simulink model "modelo_3"  (R2020a)
settings: Solver=VariableStepAuto  StartTime=0.0  StopTime=259200  RelTol=1e-3
values from neighbouring files (symbols this model uses):
  p = exp(DE/T)    [s_annealing.m]
  Pnom = 2e6    (= 2000000)    [Parametros.m]
  Pnom1 = 2e6    (= 2000000)    [Parametros.m]
  w_max = 26    [Parametros.m]
  w_min = 6    [Parametros.m]
undefined symbols (not defined in the file or in its folder): F, find_system, Fnom, gcbh, H, Llr, Lls, Rr, Rs, sps_rtmsupport, Vnom, Wind_On
libraries: powerlib x12, powerlib_meascontrol x2, re_lib x1
settings Model: Creator=octad  LastModifiedBy=octad

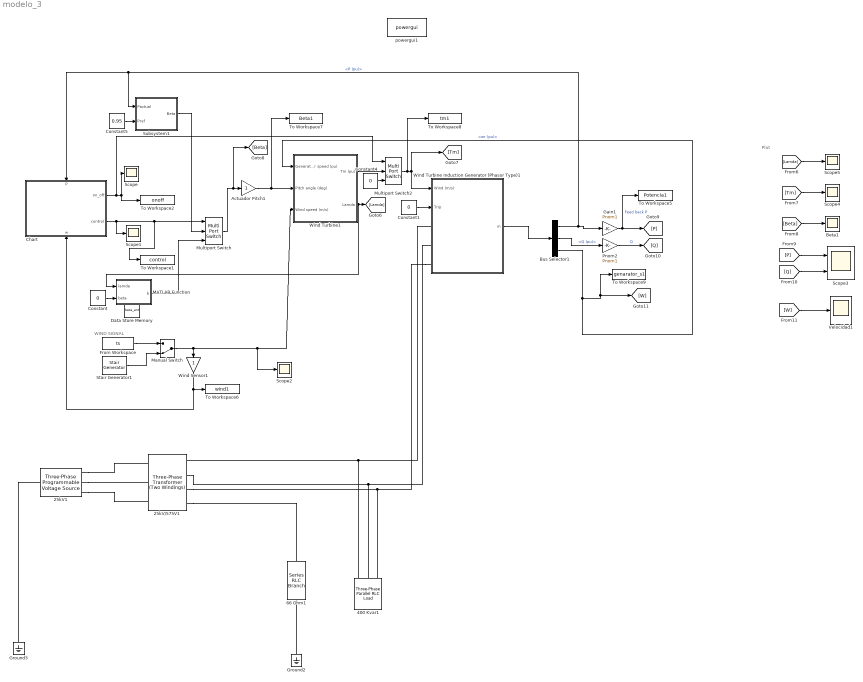
== system modelo_3 ==
  note: WIND SIGNAL
  note: Plot
  25kV/575V1 : powerlib/Elements/Three-Phase Transformer (Two Windings)  Winding1Connection=Yg  Winding2Connection=Yn  CoreType=Three single-phase transformers  SetSaturation=off  Hysteresis=off  DataFile='hysteresis'  SetInitialFlux=off  Measurements=None  UNITS=pu  NominalPower=[ 4e6 , 60 ]  Winding1=[ 25e3 , 0.025/30 , 0.025]  Winding2=[575 , 0.025/30 , 0.025 ]  Rm=500  Lm=inf  L0=0.5  Saturation=[ 0,0 ; 0.0024,1.2 ; 1.0,1.52 ]  InitialFluxes=[ 0.8 , -0.8 , 0.7 ]  BreakLoop=off  DiscreteSolver=Trapezoidal iterative  DataType=off  TransfoNumber=1
  25kV1 : powerlib/Electrical Sources/Three-Phase Programmable Voltage Source  PositiveSequence="[25000  0 60]"  VariationEntity=None  VariationType=Table of time-amplitude pairs  VariationTypeAlt=Step  VariationStep=0.5  VariationRate=10  VariationMagnitude=0.3  VariationFrequency=2  VariationTiming=[1 2]  VariationPhaseA=off  Amplitudes=[1 0.8 1.2 1.0]  TimeValues=[0 0.1 0.15 0.2]  HarmonicGeneration=off  HarmonicA=[3 0.2 -25 0]  HarmonicB=[2 0.15 35 2]  Timing="[0.05  3]"  BusType=swing  Pref=0  Qref=0  Qmin=-inf  Qmax=inf
  400 Kvar1 : powerlib/Elements/Three-Phase Parallel RLC Load  LConnTagsString=A|B|C  Configuration=Delta  NominalVoltage=575  Vabc=[1e3 1e3 1e3]  Vabcp=[1e3 1e3 1e3]  NominalFrequency=60  UnbalancedPower=off  ActivePower=0  InductivePower=0  CapacitivePower=400e3  Pabc=[10e3 9e3 11e3]  QLabc=[100 90 110]  QCabc=[100 90 110]  Pabcp=[10e3 9e3 11e3]  QLabcp=[100 90 110]  QCabcp=[100 90 110]  Measurements=None  LoadType=constant Z
  66 Ohm1 : powerlib/Elements/Series RLC Branch  LConnTagsString=__new0  RConnTagsString=__new0  BranchType=R  Resistance=66  Inductance=1e-3  SetiL0=off  InitialCurrent=0  Capacitance=1e-6  Setx0=off  InitialVoltage=0  Measurements=None
  Actuador Pitch1 : Gain
  Beta1 : Scope
  Bus Selector1 : BusSelector  OutputSignals=P (pu),Q (pu),wr (pu)
  Chart : Stateflow chart  TreatAsAtomicUnit=on
      settings: PortSchema="{\"entries\":[{\"content\":{\"sides\":[{\"content\":{\"connectorIds\":[]},\"type\":\"ConnectorPlacement.EquallySpacedRectSide\",\"uuid\":\"76455593-48be-4327-99eb-22cda1041c6c\"},{\"content\":{\"connectorIds\":[\"Out1\",\"Out2\"],\"side\":\"RIGHT\"},\"type\":\"ConnectorPlacement.EquallySpacedRectSide\",\"uuid\":\"0938c4e6-de83-48e5-b141-0954c3497832\"},{\"content\":{\"connectorIds\":[\"In2\"],\"side\":\"TOP\"},\"type\":\"ConnectorPlacement.EquallySpacedRectSide\",\"uuid\":\"886ddab1-e8c7-4b68-9a93-78c994632caa\"},{\"content\":{\"connectorIds\":[\"In1\"],\"side\":\"BOTTOM\"},\"type\":\"ConnectorPlacement.EquallySpacedRectSide\",\"uuid\":\"6af41394-77cd-4861-af48-a316959a0c75\"}]},\"type\":\"ConnectorPlacement.EquallySpacedConnector\",\"uuid\":\"704104a5-98c5-46da-8d41-4491e31041ef\"}],\"packageUris\":[\"http://schema.mathworks.com/mf0/Connector/19700101\"],\"version\":\"1.0\"}"
  Constant : Constant  Value=0
  Constant1 : Constant  Value=0
  Constant4 : Constant  Value=0
  Constant5 : Constant  Value=0.95
  Data Store Memory : DataStoreMemory  DataStoreName=beta_ant  ReadBeforeWriteMsg=warning  WriteAfterWriteMsg=warning  WriteAfterReadMsg=warning  ShowAdditionalParam=off  OutDataTypeStr=double
  From Workspace : FromWorkspace  VariableName=ts
  Gain1 : Gain  Gain=Pnom1
  Ground2 : powerlib/Elements/Ground  LConnTagsString=a
  Ground3 : powerlib/Elements/Ground  LConnTagsString=a
  MATLAB Function : MATLAB Function  TreatAsAtomicUnit=on
  Manual Switch : ManualSwitch  CurrentSetting=0
  Multiport Switch : MultiPortSwitch  DataPortOrder=Specify indices  Inputs=2  DataPortIndices={1,2}  DiagnosticForDefault=None
  Multiport Switch2 : MultiPortSwitch  DataPortOrder=Specify indices  Inputs=2  DataPortIndices={1,2}  DiagnosticForDefault=None
  Pnom2 : Gain  Gain=Pnom1
  Scope{,1..2,4..5} (5 alike) : Scope
  Scope3 : Scope  NumInputPorts=2
  Stair Generator1 : powerlib_meascontrol/Pulse & Signal Generators/Stair Generator  t=time  e=wind_d  Ts=100
  Subsystem1 : Subsystem
  To Workspace1 : ToWorkspace  VariableName=control  SaveFormat=Timeseries  SampleTime=-1
  To Workspace2 : ToWorkspace  VariableName=onoff  SaveFormat=Timeseries  SampleTime=-1
  To Workspace5 : ToWorkspace  VariableName=Potencia1  SaveFormat=Timeseries  SampleTime=-1
  To Workspace6 : ToWorkspace  VariableName=wind1  SaveFormat=Timeseries  SampleTime=-1
  To Workspace7 : ToWorkspace  VariableName=Beta1  SaveFormat=Timeseries  SampleTime=-1
  To Workspace8 : ToWorkspace  VariableName=tm1  SaveFormat=Timeseries  SampleTime=-1
  To Workspace9 : ToWorkspace  VariableName=genarator_s1  SaveFormat=Timeseries  SampleTime=-1
  Velocidad1 : Scope
  Wind Sensor1 : Gain
  Wind Turbine Induction Generator (Phasor Type)1 : Subsystem  AncestorBlock=|  DialogController=POWERSYS.PowerSysDialog  LoadFcn=sps_rtmsupport('LoadFcn',gcbh); %find_system(gcs,'FollowLinks', 'on', 'LookUnderMasks', 'all');  StartFcn=sps_rtmsupport('StartFcn',gcbh);  StopFcn=sps_rtmsupport('StopFcn',gcbh);  mask(Wind Turbine Induction Generator (Phasor Type)){ExternalTm=on, nom=[Pnom1/0.9, 575, 60], sta=[ 0.004843, 0.1248], rot=[ 0.004377, 0.1791], Lm=6.77, mec=[5.04, 0.01, 3], init=[ -0.01,0,   0,0,0,   0,0,0 ], pitch_angle=0, Pmec=1.5e6, wind_base=12, speed_nom=1, P_wind_base=1, K_pitch_gain=[5 25], pitch_max=45, pitch_rate=2}
      | re_lib/Wind Generation/Wind Turbine
      | Induction Generator
      | (Phasor Type)
      mask prompts: ExternalTm "External turbine (Tm mechanical torque input)"; nom "Nominal power, line-to-line voltage, frequency [Pn(VA), Vn(Vrms), fn(Hz)]:"; sta "Stator [Rs, Lls] (pu):"; rot "Rotor [Rr', Llr'] (pu):"; Lm "Magnetizing inductance Lm (pu):"; mec "Inertia constant, friction factor, and pairs of poles: [H(s), F(pu), p]"; init "Initial conditions [s, th(deg), ias, ibs, ics (pu), ph_as, ph_bs, ph_cs (pu)]:"; pitch_angle "Pitch angle beta used to display characteristics (beta >=0)  (deg):"; Pmec "Nominal wind turbine mechanical output power (W):"; wind_base "Base wind speed (m/s):"; speed_nom "Base rotational speed (pu of base generator speed):"; P_wind_base "Maximum power at base wind speed (pu of nominal mechanical power):"; K_pitch_gain "Pitch angle controller gain: [Kp Ki]"; pitch_max "Maximum pitch angle (deg):"; pitch_rate "Maximum rate of change of pitch angle (deg/s):"
      mask help: Implements a phasor model of a squirrel-cage induction generator driven by a wind turbine.
      mask init:
      | [Pnom,Vnom,Fnom,Rs,Lls,Rr,Llr,H,p,F,Wind_On,FACTSroot] = WindTurbineIndGenInit (nom,sta,rot,mec,ExternalTm,wind_base,gcbh);
      settings: CopyFcn=sps_rtmsupport('CopyFcn',gcbh);  DeleteFcn=sps_rtmsupport('DeleteFcn',gcbh);  UndoDeleteFcn=sps_rtmsupport('UndoDeleteFcn',gcbh);  ModelCloseFcn=sps_rtmsupport('ModelCloseFcn',gcbh);  PreSaveFcn=sps_rtmsupport('PreSaveFcn',gcbh);  PostSaveFcn=sps_rtmsupport('PostSaveFcn',gcbh);  NameChangeFcn=sps_rtmsupport('NameChangeFcn',gcbh);  PreCopyFcn=sps_rtmsupport('PreCopyFcn',gcbh);  OpenFcn=sps_rtmsupport('OpenFcn',gcbh, [1]);  CloseFcn=sps_rtmsupport('CloseFcn',gcbh);  PreDeleteFcn=sps_rtmsupport('PreDeleteFcn',gcbh);
      mask Help: helpview(psbhelp);
      mask Callback ExternalTm: WindTurbineIndGenCback(gcbh);
      mask DialogControl generatordata Prompt: Generator
      mask DialogControl Turbine Prompt: Turbine
      mask DialogControl display Prompt: Display wind turbine power characteristics
      mask DialogControl display Callback: WindTurbineIndGenDisplay(gcbh);
      mask Display:
      | image(imread(fullfile(FACTSroot,'eolienne.bmp'),'bmp'))
      | color('white')
      | port_label('LConn',1,'A')
      | port_label('LConn',2,'B')
      | port_label('LConn',3,'C')
      | color('blue')
      | port_label('output',1,'m')
      | switch get_param(gcbh,'ExternalTm')
      |     case 'on'
      |         port_label('input',1,'Tm')
      |     case 'off'
      |         port_label('input',1,'wind')
      | end
      | port_label('input',2,'trip')
  Wind Turbine1 : Subsystem  AncestorBlock=re_lib/Wind Generation/Wind Turbine  DialogController=POWERSYS.PowerSysDialog  mask(Wind Turbine){Pnom=Pnom, Pelec_base=Pnom1/0.9, wind_base=7.55, P_wind_base=0.5, speed_nom=1, pitch_angle=0, c1_c6=[0.51763          116          0.4            5           21     0.006795], cp_nom=0.48, lambda_nom=8.1}
      mask prompts: Pnom "Nominal mechanical output power (W):"; Pelec_base "Base power of the electrical generator (VA):"; wind_base "Base wind speed (m/s):"; P_wind_base "Maximum power at base wind speed (pu of nominal mechanical power):"; speed_nom "Base rotational speed (p.u. of base generator speed):"; pitch_angle "Pitch angle beta to display wind-turbine power characteristics (beta >=0)  (deg):"
      mask help:
      | This block implements a variable pitch wind turbine model. The performance coefficient Cp of the turbine is the mechanical output power of the turbine divided by wind power and a function of wind speed, rotational speed, and pitch angle (beta). Cp reaches its maximum value at zero beta. Select the wind-turbine power characteristics display to plot the turbine characteristics at the specified pitch angle.
      |
      | The first input is the generator speed in per unit of the generator base speed. For a synchronous or asynchronous generator, the base speed is the synchronous speed. For a permanent-magnet generator, the base speed is defined as the speed producing nominal voltage at  no load. The second input is the blade pitch angle (beta) in degrees. The third input is the wind speed in m/s.
      |
      | The output is the torque applied to the generator shaft in per unit of the generator ratings.
      |
      | The turbine inertia must be added to the generator inertia.
      mask init:
      | c1=c1_c6(1);c2=c1_c6(2);c3=c1_c6(3);c4=c1_c6(4);c5=c1_c6(5);c6=c1_c6(6);
      | 
      | if Pnom<=0
      |     error(message('physmod:powersys:common:GreaterThan',getfullname(gcbh),'Nominal mechanical output power',0));
      | end
      | if Pelec_base<=0
      |     error(message('physmod:powersys:common:GreaterThan',getfullname(gcbh),'Base power of the electrical generator',0));
      | end
      | if wind_base<=0
      |     error(message('physmod:powersys:common:GreaterThan',getfullname(gcbh),'Base wind speed (m/s)',0));
      | end
      | if P_wind_base<=0
      |     error(message('physmod:powersys:common:GreaterThan',getfullname(gcbh),'Maximum power at base wind speed',0));
      | end
      | power_initmask();
      settings: OpenFcn=sps_rtmsupport('OpenFcn',gcbh)
      mask Help: helpview(psbhelp);
      mask DialogControl DisplayTurbChar Prompt: Display wind turbine power characteristics
      mask DialogControl DisplayTurbChar Callback: WindTurbinePlot(gcb)
      mask Display: disp('');
  powergui1 : powerlib/powergui  Priority=1  SimulationMode=Phasor  SampleTime=50e-6  frequency=60  Iterations=50  frequencyindice=60  Pbase=100e6  ErrMax=1e-4  UnitsV=kV  UnitsW=MW  buscounter=0  FunctionMessages=off  echomessages=off  EnableUseOfTLC=off  CurrentSourceSwitches=off  DisableSnubberDevices=off  DisableRonSwitches=off  DisableVfSwitches=off  DisplayEquations=off  AutomaticDiscreteSolvers=off  SolverType=Tustin/Backward Euler (TBE)  Interpol=off  ExternalGateDelay=off  methode=off  Ts=100  x0status=blocks  SPID=on  SwTol=0  HookPort=off  NonlinearTolerance=1e-4  nMaxIteration=100  ContinueOnMaxIteration=off  RestoreLinks=warning  ResistiveCurrentMeasurement=off  Frange=[0:2:500]  Ylog=off  Xlog=on  ShowGrid=off  save=off  variable=ZData  structure=0  ZoomFFT=off  StartTime=0.0  cycles=1  DisplayStyle=1  fundamental=60  FreqAxis=off  MaxFrequency=1000  frequencyindicesteady=1  RmsSteady=1  display=off
  wires:
  Bus Selector1/1 -> Chart/2(P), Subsystem1/1(Pactual), Gain1/1  "<P (pu)>"
  Constant/1 -> MATLAB Function/2(beta)
  [Q] -> Scope3/2
  [Beta] -> Beta1/1
  Bus Selector1/2 -> Pnom2/1  "<Q (pu)>"
  Gain1/1 -> [P], To Workspace5/1  "Feed back P"
  Subsystem1/1(Beta) -> Multiport Switch/2
  Wind Turbine1/1(Tm (pu)) -> Multiport Switch2/2
  Wind Turbine Induction Generator (Phasor Type)1/1(m) -> Bus Selector1/1
  Pnom2/1 -> [Q]  "Q"
  Wind Sensor1/1 -> Chart/1(w), To Workspace6/1
  Wind Turbine1/2(Lamda) -> MATLAB Function/1(lamda), [Lamda]
  [P] -> Scope3/1
  Actuador Pitch1/1 -> To Workspace7/1, Wind Turbine1/2(Pitch angle (deg))
  [Lamda] -> Scope5/1
  [W] -> Velocidad1/1
  Constant5/1 -> Subsystem1/2(Pref)
  [Tm] -> Scope4/1
  Bus Selector1/3 -> [W], To Workspace9/1, Wind Turbine1/1(Generator speed (pu))  "<wr (pu)>"
  Multiport Switch/1 -> [Beta], Actuador Pitch1/1
  MATLAB Function/1(b) -> Multiport Switch/3
  Chart/2(control) -> Scope1/1, To Workspace1/1, Multiport Switch/1
  Chart/1(on_off) -> Multiport Switch2/1, Scope/1, To Workspace2/1
  Constant1/1 -> Wind Turbine Induction Generator (Phasor Type)1/2(Trip)
  Multiport Switch2/1 -> To Workspace8/1, [Tm], Wind Turbine Induction Generator (Phasor Type)1/1("Wind (m/s) ")
  Constant4/1 -> Multiport Switch2/3
  From Workspace/1 -> Manual Switch/1
  Stair Generator1/1 -> Manual Switch/2
  Manual Switch/1 -> Wind Sensor1/1, Scope2/1, Wind Turbine1/3(Wind speed (m/s))
  connections:
  400 Kvar1/LConn2 -- Wind Turbine Induction Generator (Phasor Type)1/LConn2 -- 25kV/575V1/RConn2
  Wind Turbine Induction Generator (Phasor Type)1/LConn3 -- 25kV/575V1/RConn3 -- 400 Kvar1/LConn3
  Wind Turbine Induction Generator (Phasor Type)1/LConn1 -- 25kV/575V1/RConn1 -- 400 Kvar1/LConn1
  25kV1/RConn1 -- 25kV/575V1/LConn1
  Ground2/LConn1 -- 66 Ohm1/RConn1
  Ground3/LConn1 -- 25kV1/LConn1
  25kV1/RConn2 -- 25kV/575V1/LConn2
  25kV/575V1/RConn4 -- 66 Ohm1/LConn1
  25kV1/RConn3 -- 25kV/575V1/LConn3

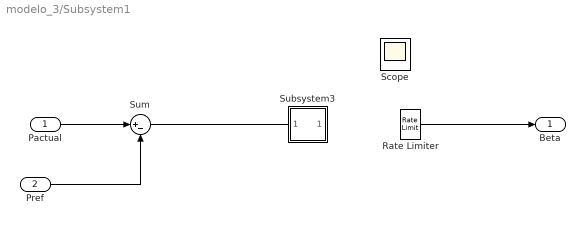
== system modelo_3/Subsystem1 ==
  Pactual : Inport
  Pref : Inport  Port=2
  "Rate Limiter   " : RateLimiter  RisingSlewLimit=2  FallingSlewLimit=-2
  Scope : Scope
  Subsystem3 : Subsystem  AncestorBlock=|  mask{Kp=1, Ki=3, Limits=[45 0], Init=0}
      | re_lib/Wind Generation/Wind Turbine
      | Induction Generator
      | (Phasor Type)/Subsystem3
      mask prompts: Kp "Proportional gain (Kp):"; Ki "Integral gain (Ki):"; Limits "Output limits [Upper Lower]:"; Init "Output initial value:"
      mask init:
      | Upper_Limit=Limits(1);
      | Lower_Limit=Limits(2);
      mask Display: disp('PI')
  Sum : Sum  Inputs=|+-
  Beta : Outport
  wires:
  Pref/1 -> Sum/2
  ? -> Scope/1, "Rate Limiter   "/1
  "Rate Limiter   "/1 -> Beta/1
  Pactual/1 -> Sum/1
  Sum/1 -> ?

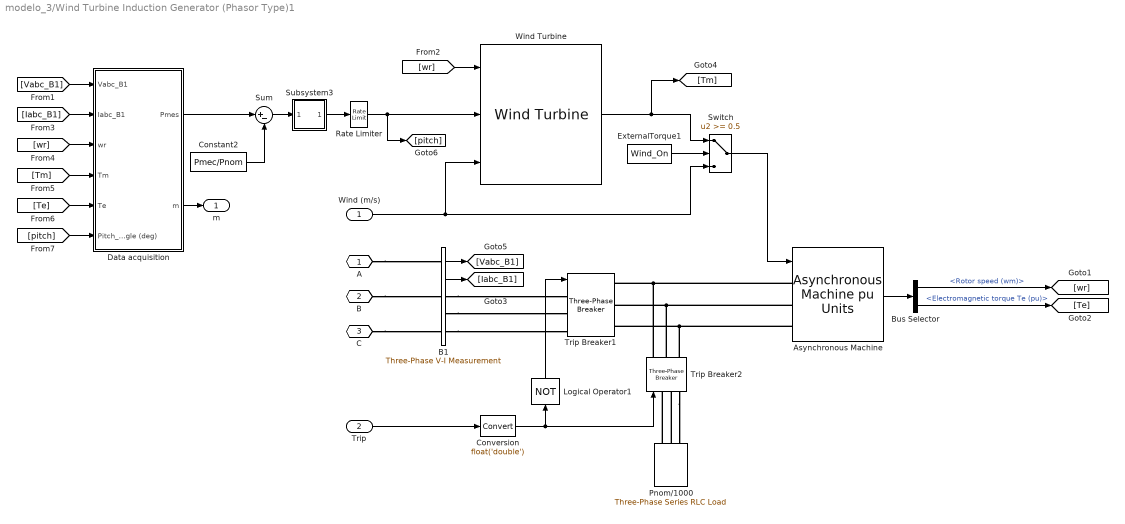
== system modelo_3/Wind Turbine Induction Generator (Phasor Type)1 ==
  "Wind (m/s) " : Inport
  Trip : Inport  Port=2
  Asynchronous Machine : powerlib/Machines/Asynchronous Machine pu Units  RotorType=Squirrel-cage  PresetModel=No  MechanicalLoad=Torque Tm  ShowDetailedParameters=on  ReferenceFrame=Rotor  Units=pu  MeasurementBus=off  NominalParameters=[ Pnom Vnom Fnom ]  Stator=[ Rs Lls]  Rotor=[ Rr Llr]  Cage1=[0.01909 0.0397]  Cage2=[0.01909 0.0397]  Lm=Lm  Mechanical=[H F p]  PolePairs=3  InitialConditions=init  SimulateSaturation=off  Saturation=[ 0 0 ; 0 0 ]  LoadFlowParameters=0  TsPowergui=0  TsBlock=-1  IterativeModel=Forward Euler  IterativeDiscreteModel=Trapezoidal non iterative  Pmec=0
      settings: SourceProductBaseCode=MT,PS
  B1 : powerlib/Measurements/Three-Phase V-I Measurement  VoltageMeasurement=phase-to-ground  SetLabelV=off  LabelV=Vabc_B1  Vpu=on  VpuLL=off  CurrentMeasurement=yes  SetLabelI=off  LabelI=Iabc_Beol  Ipu=on  Pbase=Pnom  Vbase=Vnom  OutputType=Complex  PhasorSimulation=on  PSBequivalent=0
      settings: SourceProductBaseCode=MT,PS
  Bus Selector : BusSelector  OutputSignals=Mechanical.Rotor speed (wm),Mechanical.Electromagnetic torque Te (pu)
  Constant2 : Constant  Value=Pmec/Pnom
  Conversion : DataTypeConversion  OutDataTypeStr=float('double')
  Data acquisition : Subsystem
  ExternalTorque1 : Constant  Value=Wind_On
  Logical Operator1 : Logic  Operator=NOT  AllPortsSameDT=off  OutDataTypeStr=float('double')  SampleTime=0
  Pnom/1000 : powerlib/Elements/Three-Phase Series RLC Load  LConnTagsString=A|B|C  Configuration=Y (grounded)  NominalVoltage=Vnom  Vabc=[1e3 1e3 1e3]  Vabcp=[1e3 1e3 1e3]  NominalFrequency=Fnom  UnbalancedPower=off  ActivePower=Pnom/1000  InductivePower=0  CapacitivePower=0  Pabc=[10e3 9e3 11e3]  QLabc=[100 90 110]  QCabc=[100 90 110]  Pabcp=[10e3 9e3 11e3]  QLabcp=[100 90 110]  QCabcp=[100 90 110]  Measurements=None  LoadType=constant Z
      settings: SourceProductBaseCode=MT,PS
  "Rate Limiter   " : RateLimiter  RisingSlewLimit=pitch_rate  FallingSlewLimit=-pitch_rate
  Subsystem3 : Subsystem  mask{Kp=K_pitch_gain(1), Ki=K_pitch_gain(2), Limits=[pitch_max 0], Init=0}
      mask prompts: Kp "Proportional gain (Kp):"; Ki "Integral gain (Ki):"; Limits "Output limits [Upper Lower]:"; Init "Output initial value:"
      mask init:
      | Upper_Limit=Limits(1);
      | Lower_Limit=Limits(2);
      mask Display: disp('PI')
  Sum : Sum  Inputs=|+-  SaturateOnIntegerOverflow=on
  Switch : Switch  Threshold=0.5  SaturateOnIntegerOverflow=on
  Trip Breaker1 : powerlib/Elements/Three-Phase Breaker  InitialState=closed  SwitchA=on  SwitchB=on  SwitchC=on  SwitchTimes="[4/60  10/60]"  External=on  BreakerResistance=0.001  SnubberResistance=1e6  SnubberCapacitance=inf  Measurements=None
      settings: SourceProductBaseCode=MT,PS
  Trip Breaker2 : powerlib/Elements/Three-Phase Breaker  InitialState=open  SwitchA=on  SwitchB=on  SwitchC=on  SwitchTimes="[4/60  10/60]"  External=on  BreakerResistance=0.001  SnubberResistance=1e6  SnubberCapacitance=inf  Measurements=None
      settings: SourceProductBaseCode=MT,PS
  Wind Turbine : re_lib/Wind Generation/Wind Turbine  Pnom=Pmec  Pelec_base=Pnom  wind_base=wind_base  P_wind_base=P_wind_base  speed_nom=speed_nom  pitch_angle=0  c1_c6="[0.51763          116          0.4            5           21     0.006795]"  cp_nom=0.48  lambda_nom=8.1
      settings: SourceProductBaseCode=PS
  A : PMIOPort  Side=Left
  B : PMIOPort  Port=2  Side=Left
  C : PMIOPort  Port=3  Side=Left
  m : Outport  VectorParamsAs1DForOutWhenUnconnected=off
  wires:
  Asynchronous Machine/1 -> Bus Selector/1
  Wind Turbine/1 -> Switch/1, [Tm]
  B1/2 -> [Iabc_B1]
  B1/1 -> [Vabc_B1]
  "Wind (m/s) "/1 -> Wind Turbine/3, Switch/3
  Data acquisition/2(m) -> m/1
  "Rate Limiter   "/1 -> Wind Turbine/2, [pitch]
  Bus Selector/1 -> [wr]  "<Rotor speed (wm)>"
  Bus Selector/2 -> [Te]  "<Electromagnetic torque Te (pu)>"
  [Iabc_B1] -> Data acquisition/2(Iabc_B1)
  [Vabc_B1] -> Data acquisition/1(Vabc_B1)
  [wr] -> Data acquisition/3(wr)
  [Tm] -> Data acquisition/4(Tm)
  [Te] -> Data acquisition/5(Te)
  [pitch] -> Data acquisition/6(Pitch_angle (deg))
  Trip/1 -> Conversion/1
  ExternalTorque1/1 -> Switch/2
  Switch/1 -> Asynchronous Machine/1
  Sum/1 -> Subsystem3/1(In1)
  Subsystem3/1(Out1) -> "Rate Limiter   "/1
  Constant2/1 -> Sum/2
  Conversion/1 -> Logical Operator1/1, Trip Breaker2/1
  Logical Operator1/1 -> Trip Breaker1/1
  Data acquisition/1(Pmes) -> Sum/1
  [wr] -> Wind Turbine/1
  connections:
  Trip Breaker2/LConn3 -- Pnom/1000/LConn3
  B1/RConn3 -- Trip Breaker1/LConn3
  B/RConn1 -- B1/LConn2
  C/RConn1 -- B1/LConn3
  A/RConn1 -- B1/LConn1
  Trip Breaker2/RConn1 -- Trip Breaker1/RConn1 -- Asynchronous Machine/LConn1
  Trip Breaker2/RConn2 -- Trip Breaker1/RConn2 -- Asynchronous Machine/LConn2
  Trip Breaker2/RConn3 -- Trip Breaker1/RConn3 -- Asynchronous Machine/LConn3
  B1/RConn1 -- Trip Breaker1/LConn1
  B1/RConn2 -- Trip Breaker1/LConn2
  Pnom/1000/LConn1 -- Trip Breaker2/LConn1
  Pnom/1000/LConn2 -- Trip Breaker2/LConn2

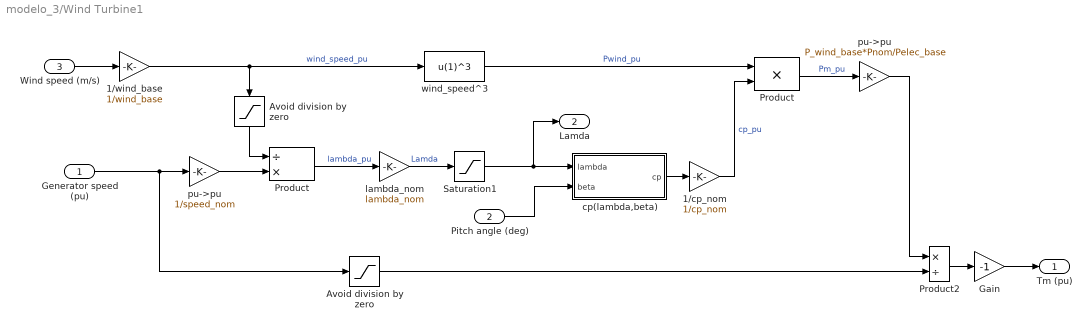
== system modelo_3/Wind Turbine1 ==
  Generator speed (pu) : Inport
  Pitch angle (deg) : Inport  Port=2
  Wind speed (m/s) : Inport  Port=3
  1/cp_nom : Gain  Gain=1/cp_nom  SaturateOnIntegerOverflow=on  OutDataTypeStr=Inherit: Same as input  ParamDataTypeStr=Inherit: Same as input
  1/wind_base : Gain  Gain=1/wind_base  SaturateOnIntegerOverflow=on  OutDataTypeStr=Inherit: Same as input  ParamDataTypeStr=Inherit: Same as input
  Avoid division by zero : Saturate  UpperLimit=1e6  LowerLimit=1e-6
  "Avoid division by zero " : Saturate  UpperLimit=inf  LowerLimit=1e-6
  Gain : Gain  Gain=-1  SaturateOnIntegerOverflow=on  OutDataTypeStr=Inherit: Same as input  ParamDataTypeStr=Inherit: Same as input
  Product : Product  Inputs=/*  SaturateOnIntegerOverflow=on  OutDataTypeStr=Inherit: Same as first input
  "Product " : Product  SaturateOnIntegerOverflow=on  OutDataTypeStr=Inherit: Same as first input
  Product2 : Product  Inputs=*/  InputSameDT=on  SaturateOnIntegerOverflow=on  OutDataTypeStr=Inherit: Same as first input
  Saturation1 : Saturate  UpperLimit=inf  LowerLimit=1e-6
  cp(lambda,beta) : Subsystem
  lambda_nom : Gain  Gain=lambda_nom  SaturateOnIntegerOverflow=on  OutDataTypeStr=Inherit: Same as input  ParamDataTypeStr=Inherit: Same as input
  pu->pu : Gain  Gain=P_wind_base*Pnom/Pelec_base  SaturateOnIntegerOverflow=on  OutDataTypeStr=Inherit: Same as input  ParamDataTypeStr=Inherit: Same as input
  "pu->pu " : Gain  Gain=1/speed_nom  SaturateOnIntegerOverflow=on  OutDataTypeStr=Inherit: Same as input  ParamDataTypeStr=Inherit: Same as input
  wind_speed^3 : Fcn  Expr=u(1)^3
  Tm (pu) : Outport  VectorParamsAs1DForOutWhenUnconnected=off
  Lamda : Outport  Port=2
  wires:
  Pitch angle (deg)/1 -> cp(lambda,beta)/2(beta)
  pu->pu/1 -> Product2/1
  cp(lambda,beta)/1(cp) -> 1/cp_nom/1
  wind_speed^3/1 -> "Product "/1  "Pwind_pu"
  Product2/1 -> Gain/1
  Avoid division by zero/1 -> Product2/2
  Wind speed (m/s)/1 -> 1/wind_base/1
  Gain/1 -> Tm (pu)/1
  Generator speed (pu)/1 -> Avoid division by zero/1, "pu->pu "/1
  "Product "/1 -> pu->pu/1  "Pm_pu"
  lambda_nom/1 -> Saturation1/1  "Lamda"
  1/cp_nom/1 -> "Product "/2  "cp_pu"
  Saturation1/1 -> cp(lambda,beta)/1(lambda), Lamda/1
  Product/1 -> lambda_nom/1  "lambda_pu"
  1/wind_base/1 -> wind_speed^3/1, "Avoid division by zero "/1  "wind_speed_pu"
  "Avoid division by zero "/1 -> Product/1
  "pu->pu "/1 -> Product/2

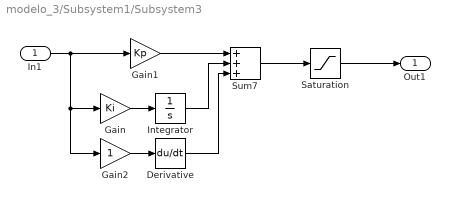
== system modelo_3/Subsystem1/Subsystem3 ==
  In1 : Inport
  Derivative : Derivative
  Gain : Gain  Gain=Ki  SaturateOnIntegerOverflow=on  OutDataTypeStr=Inherit: Same as input  ParamDataTypeStr=Inherit: Same as input
  Gain1 : Gain  Gain=Kp  SaturateOnIntegerOverflow=on  OutDataTypeStr=Inherit: Same as input  ParamDataTypeStr=Inherit: Same as input
  Gain2 : Gain
  Integrator : Integrator  InitialCondition=Init  LimitOutput=on  UpperSaturationLimit=Upper_Limit  LowerSaturationLimit=Lower_Limit
  Saturation : Saturate  UpperLimit=Upper_Limit  LowerLimit=Lower_Limit
  Sum7 : Sum  Inputs=+++  InputSameDT=on  SaturateOnIntegerOverflow=on  OutDataTypeStr=Inherit: Same as first input
  Out1 : Outport  VectorParamsAs1DForOutWhenUnconnected=off
  wires:
  Gain/1 -> Integrator/1
  Gain1/1 -> Sum7/1
  Gain2/1 -> Derivative/1
  Derivative/1 -> Sum7/3
  Integrator/1 -> Sum7/2
  Saturation/1 -> Out1/1
  In1/1 -> Gain2/1, Gain/1, Gain1/1
  Sum7/1 -> Saturation/1

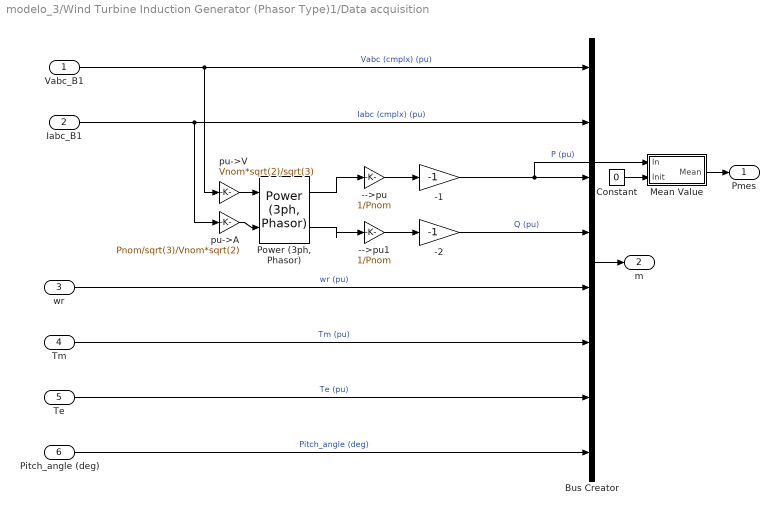
== system modelo_3/Wind Turbine Induction Generator (Phasor Type)1/Data acquisition ==
  Vabc_B1 : Inport
  Iabc_B1 : Inport  Port=2
  wr : Inport  Port=3
  Tm : Inport  Port=4
  Te : Inport  Port=5
  Pitch_angle (deg) : Inport  Port=6
  -->pu : Gain  Gain=1/Pnom  SaturateOnIntegerOverflow=on  OutDataTypeStr=Inherit: Same as input  ParamDataTypeStr=Inherit: Same as input
  -->pu1 : Gain  Gain=1/Pnom  SaturateOnIntegerOverflow=on  OutDataTypeStr=Inherit: Same as input  ParamDataTypeStr=Inherit: Same as input
  -1 : Gain  Gain=-1  SaturateOnIntegerOverflow=on  OutDataTypeStr=Inherit: Same as input  ParamDataTypeStr=Inherit: Same as input
  -2 : Gain  Gain=-1  SaturateOnIntegerOverflow=on  OutDataTypeStr=Inherit: Same as input  ParamDataTypeStr=Inherit: Same as input
  Bus Creator : BusCreator  Inputs=8
  Constant : Constant  Value=0
  Mean Value : Subsystem  mask(Mean value){Period=1/Fnom}
      mask prompts: Period "Averaging period (s):"
      mask help: This block uses the running window averaging technique to compute the mean value of the input signal over the specified period.
  "Power (3ph, Phasor)" : powerlib_meascontrol/Measurements/Power (3ph, Phasor)
      settings: SourceProductBaseCode=MT,PS
  pu->A : Gain  Gain=Pnom/sqrt(3)/Vnom*sqrt(2)  SaturateOnIntegerOverflow=on  OutDataTypeStr=Inherit: Same as input  ParamDataTypeStr=Inherit: Same as input
  pu->V : Gain  Gain=Vnom*sqrt(2)/sqrt(3)  SaturateOnIntegerOverflow=on  OutDataTypeStr=Inherit: Same as input  ParamDataTypeStr=Inherit: Same as input
  Pmes : Outport  VectorParamsAs1DForOutWhenUnconnected=off
  m : Outport  Port=2  VectorParamsAs1DForOutWhenUnconnected=off
  wires:
  "Power (3ph, Phasor)"/2 -> -->pu1/1
  "Power (3ph, Phasor)"/1 -> -->pu/1
  -->pu1/1 -> -2/1
  Bus Creator/1 -> m/1
  Mean Value/1(Mean) -> Pmes/1
  Constant/1 -> Mean Value/2(Init)
  Iabc_B1/1 -> Bus Creator/2, pu->A/1  "Iabc (cmplx) (pu)"
  Vabc_B1/1 -> Bus Creator/1, pu->V/1  "Vabc (cmplx) (pu)"
  Pitch_angle (deg)/1 -> Bus Creator/8  "Pitch_angle (deg)"
  Te/1 -> Bus Creator/7  "Te (pu)"
  Tm/1 -> Bus Creator/6  "Tm (pu)"
  wr/1 -> Bus Creator/5  "wr (pu)"
  -1/1 -> Bus Creator/3, Mean Value/1(In)  "P (pu)"
  -2/1 -> Bus Creator/4  "Q (pu)"
  pu->V/1 -> "Power (3ph, Phasor)"/1
  -->pu/1 -> -1/1
  pu->A/1 -> "Power (3ph, Phasor)"/2

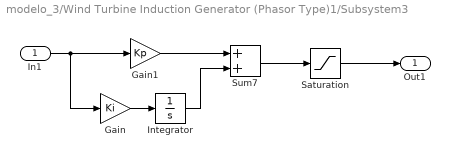
== system modelo_3/Wind Turbine Induction Generator (Phasor Type)1/Subsystem3 ==
  In1 : Inport
  Gain : Gain  Gain=Ki  SaturateOnIntegerOverflow=on  OutDataTypeStr=Inherit: Same as input  ParamDataTypeStr=Inherit: Same as input
  Gain1 : Gain  Gain=Kp  SaturateOnIntegerOverflow=on  OutDataTypeStr=Inherit: Same as input  ParamDataTypeStr=Inherit: Same as input
  Integrator : Integrator  InitialCondition=Init  LimitOutput=on  UpperSaturationLimit=Upper_Limit  LowerSaturationLimit=Lower_Limit
  Saturation : Saturate  UpperLimit=Upper_Limit  LowerLimit=Lower_Limit
  Sum7 : Sum  InputSameDT=on  SaturateOnIntegerOverflow=on  OutDataTypeStr=Inherit: Same as first input
  Out1 : Outport  VectorParamsAs1DForOutWhenUnconnected=off
  wires:
  Saturation/1 -> Out1/1
  Sum7/1 -> Saturation/1
  In1/1 -> Gain/1, Gain1/1
  Integrator/1 -> Sum7/2
  Gain1/1 -> Sum7/1
  Gain/1 -> Integrator/1

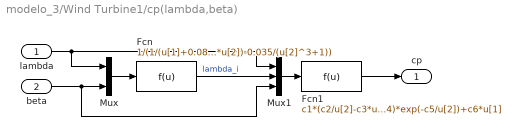
== system modelo_3/Wind Turbine1/cp(lambda,beta) ==
  lambda : Inport
  beta : Inport  Port=2
  Fcn : Fcn  Expr=1/(1/(u[1]+0.08*u[2])-0.035/(u[2]^3+1))
  Fcn1 : Fcn  Expr=c1*(c2/u[2]-c3*u[3]-c4)*exp(-c5/u[2])+c6*u[1]
  Mux : Mux  Inputs=2
  Mux1 : Mux  Inputs=3
  cp : Outport  VectorParamsAs1DForOutWhenUnconnected=off
  wires:
  Fcn/1 -> Mux1/2  "lambda_i"
  Fcn1/1 -> cp/1
  lambda/1 -> Mux1/1, Mux/1
  Mux1/1 -> Fcn1/1
  beta/1 -> Mux1/3, Mux/2
  Mux/1 -> Fcn/1

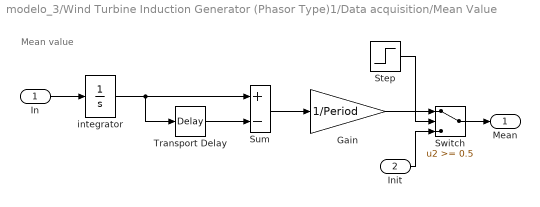
== system modelo_3/Wind Turbine Induction Generator (Phasor Type)1/Data acquisition/Mean Value ==
  note: Mean value
  In : Inport
  Init : Inport  Port=2
  Gain : Gain  Gain=1/Period  SaturateOnIntegerOverflow=on  OutDataTypeStr=Inherit: Same as input  ParamDataTypeStr=Inherit: Same as input
  Step : Step  Time=Period+eps  SampleTime=0
  Sum : Sum  Inputs=+-  InputSameDT=on  SaturateOnIntegerOverflow=on  OutDataTypeStr=Inherit: Same as first input
  Switch : Switch  Threshold=0.5  SaturateOnIntegerOverflow=on
  Transport Delay : TransportDelay  DelayTime=Period
  integrator : Integrator
  Mean : Outport  VectorParamsAs1DForOutWhenUnconnected=off
  wires:
  Transport Delay/1 -> Sum/2
  integrator/1 -> Transport Delay/1, Sum/1
  In/1 -> integrator/1
  Sum/1 -> Gain/1
  Gain/1 -> Switch/1
  Switch/1 -> Mean/1
  Step/1 -> Switch/2
  Init/1 -> Switch/3

== matlab function modelo_3/MATLAB Function ==
  settings: updateMethod=DISCRETE
  data: lamda input; b output; beta input; beta_ant data_store_memory
function b = fcn(lamda, beta)
global beta_ant;

b= s_annealing(lamda, beta);
beta_ant=b;
end

== stateflow chart modelo_3/Chart ==
  state T_OFF
    entry: on_off=2;
    entry: control=1;
  state T_ON
    entry: on_off=1;
    state s_a
      entry: control=2;
    state p_i
      entry: control=1;
    (default) -> s_a
    s_a -> p_i : [w>=17]
    p_i -> s_a : [w<17]
  (default) -> T_OFF
  T_OFF -> T_ON : [w<w_max & w>w_min]
  T_ON -> T_OFF : [w>w_max || w<w_min]
  data: w_max parameter; w input; w_min parameter; on_off output; control output; P input
